simulink model "Controller"  (R2024b)
settings: Solver=VariableStepAuto  StartTime=0.0  StopTime=45  FixedStep=0.001  RelTol=1e-3
undefined symbols (not defined in the file): K_W, kd, ki, kp, tl, u_bar_max
settings Model: Creator=Enrico  LastModifiedBy=farin
settings DataIOCC: ReturnWorkspaceOutputsName=out_black_box

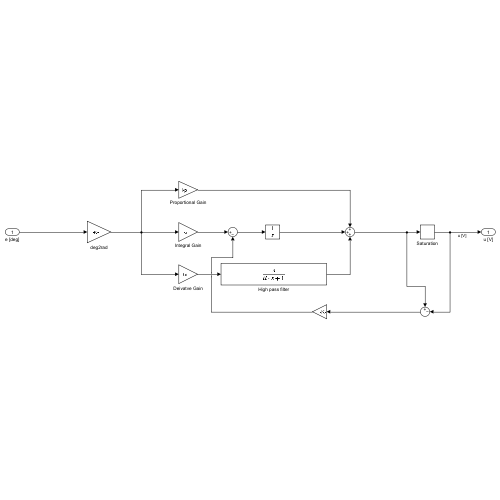
[thumbnail: Simulink's stored preview of the top-level diagram]
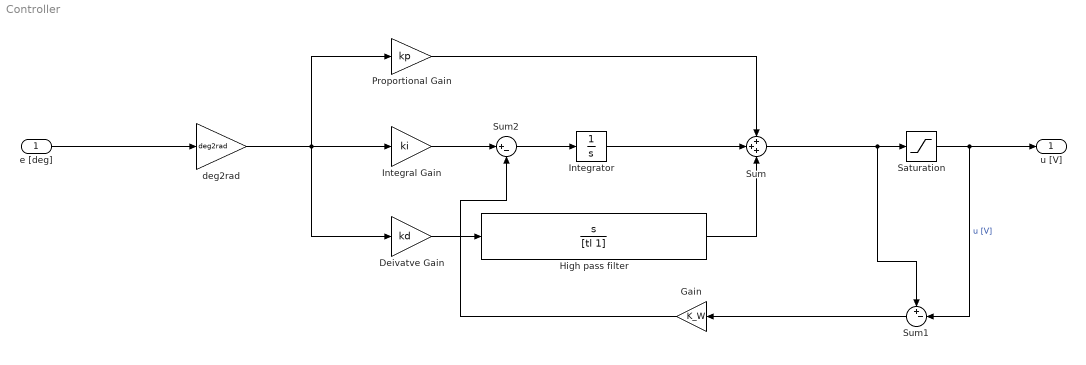
== system Controller ==
  e [deg] : Inport
  Deivatve Gain : Gain  Gain=kd
  Gain : Gain  Gain=K_W
  High pass filter : TransferFcn  Numerator=[1 0]  Denominator=[tl 1]
  Integral Gain : Gain  Gain=ki
  Integrator : Integrator
  Proportional Gain : Gain  Gain=kp
  "Saturation " : Saturate  UpperLimit=u_bar_max  LowerLimit=-u_bar_max
  Sum : Sum  Inputs=+++
  Sum1 : Sum  Inputs=+-|
  Sum2 : Sum  Inputs=|+-
  deg2rad : Gain  Gain=deg2rad
  u [V] : Outport
  wires:
  Deivatve Gain/1 -> High pass filter/1
  Sum1/1 -> Gain/1
  Proportional Gain/1 -> Sum/1
  e [deg]/1 -> deg2rad/1
  Sum2/1 -> Integrator/1
  Sum/1 -> Sum1/1, "Saturation "/1
  High pass filter/1 -> Sum/3
  Integrator/1 -> Sum/2
  deg2rad/1 -> Deivatve Gain/1, Proportional Gain/1, Integral Gain/1
  Gain/1 -> Sum2/2
  "Saturation "/1 -> Sum1/2, u [V]/1  "u [V]"
  Integral Gain/1 -> Sum2/1
